simulink model "Pokus07_Display"  (Simulink 8.1)
settings: Solver=ode45  StartTime=0.0  StopTime=10.0  RelTol=1e-3
undefined symbols (not defined in the file): A, ARROW_DOWN, ARROW_LEFT, ARROW_RIGHT, ARROW_UP, ASTERISK, B, BACKSLASH, C, COLON, COMMA, CROSS, CURSOR, D, DOT, ending_column_index, ending_row_index, EQUAL, EXCLAMATION_MARK, F, framebuffer, G, GREATER_THAN, H, HEIGHT, hot, I, J, K, L, LEFT_PARENTHESES, LESS_THAN, M, MINUS, N, O, P, PERCENT, PLUS, POS_X, POS_Y, Q, QUESTION_MARK, QUOTE, R, RECTANGLE, RIGHT_PARENTHESES, S, SEMICOLON, SHARP, SLASH, SPACE, starting_column_index, starting_row_index, T, U, UNDERSCORE, V, W, WIDTH ... (+6)
libraries: dspmtrx3 x197, Common_Library x69, commutil2 x53, simulink_extras x1, dspsnks4 x1
(part 3 of 6)

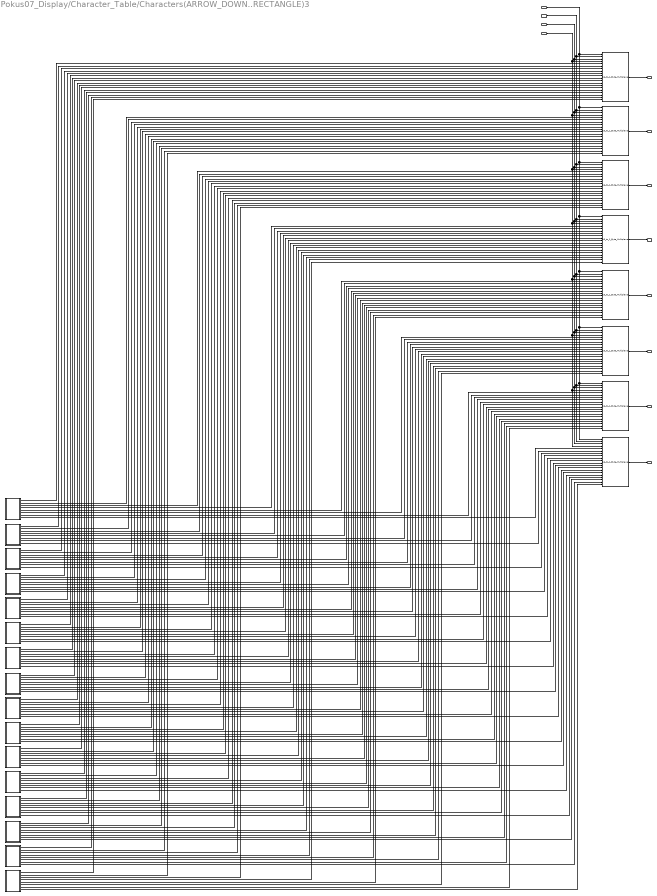
== system Pokus07_Display/Character_Table/Characters(ARROW_DOWN..RECTANGLE)3 ==
  Address_3_In(1b) : Inport
  Address_2_In(1b) : Inport  Port=2
  Address_1_In(1b) : Inport  Port=3
  Address_0_In(1b) : Inport  Port=4
  16_to_1_Byte_Multiplexer{,1..7} (8 alike) : Common_Library/Multiplexers/16_to_1_Byte_Multiplexer
  Char_ARROW_DOWN : Subsystem
  Char_ARROW_LEFT : Subsystem
  Char_ARROW_RIGHT : Subsystem
  Char_COMMA : Subsystem
  Char_CURSOR : Subsystem
  Char_DOT : Subsystem
  Char_EXCLAMATION_MARK : Subsystem
  Char_LEFT_PARENTHESES : Subsystem
  Char_PERCENT : Subsystem
  Char_QUESTION_MARK : Subsystem
  Char_QUOTE : Subsystem
  Char_RECTANGLE : Subsystem
  Char_RIGHT_PARENTHESES : Subsystem
  Char_SHARP : Subsystem
  Char_SPACE : Subsystem
  Char_UNDERSCORE : Subsystem
  Column_1(1B) : Outport
  Column_2(1B) : Outport  Port=2
  Column_3(1B) : Outport  Port=3
  Column_4(1B) : Outport  Port=4
  Column_5(1B) : Outport  Port=5
  Column_6(1B) : Outport  Port=6
  Column_7(1B) : Outport  Port=7
  Column_8(1B) : Outport  Port=8
  wires:
  Char_RECTANGLE/1(Column_1(1B)) -> 16_to_1_Byte_Multiplexer/5
  Char_CURSOR/1(Column_1(1B)) -> 16_to_1_Byte_Multiplexer/6
  Char_SPACE/1(Column_1(1B)) -> 16_to_1_Byte_Multiplexer/7
  Char_RIGHT_PARENTHESES/1(Column_1(1B)) -> 16_to_1_Byte_Multiplexer/8
  Char_LEFT_PARENTHESES/1(Column_1(1B)) -> 16_to_1_Byte_Multiplexer/9
  Char_PERCENT/1(Column_1(1B)) -> 16_to_1_Byte_Multiplexer/10
  Char_SHARP/1(Column_1(1B)) -> 16_to_1_Byte_Multiplexer/11
  Char_QUOTE/1(Column_1(1B)) -> 16_to_1_Byte_Multiplexer/12
  Char_EXCLAMATION_MARK/1(Column_1(1B)) -> 16_to_1_Byte_Multiplexer/13
  Char_QUESTION_MARK/1(Column_1(1B)) -> 16_to_1_Byte_Multiplexer/14
  Char_COMMA/1(Column_1(1B)) -> 16_to_1_Byte_Multiplexer/15
  Char_DOT/1(Column_1(1B)) -> 16_to_1_Byte_Multiplexer/16
  Char_UNDERSCORE/1(Column_1(1B)) -> 16_to_1_Byte_Multiplexer/17
  Char_ARROW_RIGHT/1(Column_1(1B)) -> 16_to_1_Byte_Multiplexer/18
  Char_ARROW_LEFT/1(Column_1(1B)) -> 16_to_1_Byte_Multiplexer/19
  Char_ARROW_DOWN/1(Column_1(1B)) -> 16_to_1_Byte_Multiplexer/20
  Char_RECTANGLE/2(Column_2(1B)) -> 16_to_1_Byte_Multiplexer1/5
  Char_ARROW_DOWN/2(Column_2(1B)) -> 16_to_1_Byte_Multiplexer1/20
  Char_ARROW_LEFT/2(Column_2(1B)) -> 16_to_1_Byte_Multiplexer1/19
  Char_ARROW_RIGHT/2(Column_2(1B)) -> 16_to_1_Byte_Multiplexer1/18
  Char_UNDERSCORE/2(Column_2(1B)) -> 16_to_1_Byte_Multiplexer1/17
  Char_DOT/2(Column_2(1B)) -> 16_to_1_Byte_Multiplexer1/16
  Char_COMMA/2(Column_2(1B)) -> 16_to_1_Byte_Multiplexer1/15
  Char_QUESTION_MARK/2(Column_2(1B)) -> 16_to_1_Byte_Multiplexer1/14
  Char_EXCLAMATION_MARK/2(Column_2(1B)) -> 16_to_1_Byte_Multiplexer1/13
  Char_QUOTE/2(Column_2(1B)) -> 16_to_1_Byte_Multiplexer1/12
  Char_SHARP/2(Column_2(1B)) -> 16_to_1_Byte_Multiplexer1/11
  Char_PERCENT/2(Column_2(1B)) -> 16_to_1_Byte_Multiplexer1/10
  Char_LEFT_PARENTHESES/2(Column_2(1B)) -> 16_to_1_Byte_Multiplexer1/9
  Char_RIGHT_PARENTHESES/2(Column_2(1B)) -> 16_to_1_Byte_Multiplexer1/8
  Char_SPACE/2(Column_2(1B)) -> 16_to_1_Byte_Multiplexer1/7
  Char_CURSOR/2(Column_2(1B)) -> 16_to_1_Byte_Multiplexer1/6
  Char_ARROW_DOWN/3(Column_3(1B)) -> 16_to_1_Byte_Multiplexer2/20
  Char_ARROW_LEFT/3(Column_3(1B)) -> 16_to_1_Byte_Multiplexer2/19
  Char_ARROW_RIGHT/3(Column_3(1B)) -> 16_to_1_Byte_Multiplexer2/18
  Char_UNDERSCORE/3(Column_3(1B)) -> 16_to_1_Byte_Multiplexer2/17
  Char_DOT/3(Column_3(1B)) -> 16_to_1_Byte_Multiplexer2/16
  Char_COMMA/3(Column_3(1B)) -> 16_to_1_Byte_Multiplexer2/15
  Char_QUESTION_MARK/3(Column_3(1B)) -> 16_to_1_Byte_Multiplexer2/14
  Char_EXCLAMATION_MARK/3(Column_3(1B)) -> 16_to_1_Byte_Multiplexer2/13
  Char_QUOTE/3(Column_3(1B)) -> 16_to_1_Byte_Multiplexer2/12
  Char_SHARP/3(Column_3(1B)) -> 16_to_1_Byte_Multiplexer2/11
  Char_PERCENT/3(Column_3(1B)) -> 16_to_1_Byte_Multiplexer2/10
  Char_LEFT_PARENTHESES/3(Column_3(1B)) -> 16_to_1_Byte_Multiplexer2/9
  Char_RIGHT_PARENTHESES/3(Column_3(1B)) -> 16_to_1_Byte_Multiplexer2/8
  Char_SPACE/3(Column_3(1B)) -> 16_to_1_Byte_Multiplexer2/7
  Char_CURSOR/3(Column_3(1B)) -> 16_to_1_Byte_Multiplexer2/6
  Char_RECTANGLE/3(Column_3(1B)) -> 16_to_1_Byte_Multiplexer2/5
  Char_ARROW_DOWN/4(Column_4(1B)) -> 16_to_1_Byte_Multiplexer3/20
  Char_ARROW_LEFT/4(Column_4(1B)) -> 16_to_1_Byte_Multiplexer3/19
  Char_ARROW_RIGHT/4(Column_4(1B)) -> 16_to_1_Byte_Multiplexer3/18
  Char_UNDERSCORE/4(Column_4(1B)) -> 16_to_1_Byte_Multiplexer3/17
  Char_DOT/4(Column_4(1B)) -> 16_to_1_Byte_Multiplexer3/16
  Char_COMMA/4(Column_4(1B)) -> 16_to_1_Byte_Multiplexer3/15
  Char_QUESTION_MARK/4(Column_4(1B)) -> 16_to_1_Byte_Multiplexer3/14
  Char_EXCLAMATION_MARK/4(Column_4(1B)) -> 16_to_1_Byte_Multiplexer3/13
  Char_QUOTE/4(Column_4(1B)) -> 16_to_1_Byte_Multiplexer3/12
  Char_SHARP/4(Column_4(1B)) -> 16_to_1_Byte_Multiplexer3/11
  Char_PERCENT/4(Column_4(1B)) -> 16_to_1_Byte_Multiplexer3/10
  Char_LEFT_PARENTHESES/4(Column_4(1B)) -> 16_to_1_Byte_Multiplexer3/9
  Char_RIGHT_PARENTHESES/4(Column_4(1B)) -> 16_to_1_Byte_Multiplexer3/8
  Char_SPACE/4(Column_4(1B)) -> 16_to_1_Byte_Multiplexer3/7
  Char_CURSOR/4(Column_4(1B)) -> 16_to_1_Byte_Multiplexer3/6
  Char_RECTANGLE/4(Column_4(1B)) -> 16_to_1_Byte_Multiplexer3/5
  Char_ARROW_DOWN/5(Column_5(1B)) -> 16_to_1_Byte_Multiplexer4/20
  Char_ARROW_LEFT/5(Column_5(1B)) -> 16_to_1_Byte_Multiplexer4/19
  Char_ARROW_RIGHT/5(Column_5(1B)) -> 16_to_1_Byte_Multiplexer4/18
  Char_UNDERSCORE/5(Column_5(1B)) -> 16_to_1_Byte_Multiplexer4/17
  Char_DOT/5(Column_5(1B)) -> 16_to_1_Byte_Multiplexer4/16
  Char_COMMA/5(Column_5(1B)) -> 16_to_1_Byte_Multiplexer4/15
  Char_EXCLAMATION_MARK/5(Column_5(1B)) -> 16_to_1_Byte_Multiplexer4/13
  Char_QUESTION_MARK/5(Column_5(1B)) -> 16_to_1_Byte_Multiplexer4/14
  Char_QUOTE/5(Column_5(1B)) -> 16_to_1_Byte_Multiplexer4/12
  Char_SHARP/5(Column_5(1B)) -> 16_to_1_Byte_Multiplexer4/11
  Char_PERCENT/5(Column_5(1B)) -> 16_to_1_Byte_Multiplexer4/10
  Char_LEFT_PARENTHESES/5(Column_5(1B)) -> 16_to_1_Byte_Multiplexer4/9
  Char_RIGHT_PARENTHESES/5(Column_5(1B)) -> 16_to_1_Byte_Multiplexer4/8
  Char_SPACE/5(Column_5(1B)) -> 16_to_1_Byte_Multiplexer4/7
  Char_CURSOR/5(Column_5(1B)) -> 16_to_1_Byte_Multiplexer4/6
  Char_RECTANGLE/5(Column_5(1B)) -> 16_to_1_Byte_Multiplexer4/5
  Char_ARROW_DOWN/6(Column_6(1B)) -> 16_to_1_Byte_Multiplexer5/20
  Char_ARROW_LEFT/6(Column_6(1B)) -> 16_to_1_Byte_Multiplexer5/19
  Char_ARROW_RIGHT/6(Column_6(1B)) -> 16_to_1_Byte_Multiplexer5/18
  Char_UNDERSCORE/6(Column_6(1B)) -> 16_to_1_Byte_Multiplexer5/17
  Char_DOT/6(Column_6(1B)) -> 16_to_1_Byte_Multiplexer5/16
  Char_COMMA/6(Column_6(1B)) -> 16_to_1_Byte_Multiplexer5/15
  Char_QUESTION_MARK/6(Column_6(1B)) -> 16_to_1_Byte_Multiplexer5/14
  Char_EXCLAMATION_MARK/6(Column_6(1B)) -> 16_to_1_Byte_Multiplexer5/13
  Char_QUOTE/6(Column_6(1B)) -> 16_to_1_Byte_Multiplexer5/12
  Char_SHARP/6(Column_6(1B)) -> 16_to_1_Byte_Multiplexer5/11
  Char_PERCENT/6(Column_6(1B)) -> 16_to_1_Byte_Multiplexer5/10
  Char_LEFT_PARENTHESES/6(Column_6(1B)) -> 16_to_1_Byte_Multiplexer5/9
  Char_RIGHT_PARENTHESES/7(Column_7(1B)) -> 16_to_1_Byte_Multiplexer6/8
  Char_RIGHT_PARENTHESES/6(Column_6(1B)) -> 16_to_1_Byte_Multiplexer5/8
  Char_SPACE/6(Column_6(1B)) -> 16_to_1_Byte_Multiplexer5/7
  Char_CURSOR/6(Column_6(1B)) -> 16_to_1_Byte_Multiplexer5/6
  Char_RECTANGLE/6(Column_6(1B)) -> 16_to_1_Byte_Multiplexer5/5
  Char_ARROW_DOWN/7(Column_7(1B)) -> 16_to_1_Byte_Multiplexer6/20
  Char_ARROW_LEFT/7(Column_7(1B)) -> 16_to_1_Byte_Multiplexer6/19
  Char_ARROW_RIGHT/7(Column_7(1B)) -> 16_to_1_Byte_Multiplexer6/18
  Char_UNDERSCORE/7(Column_7(1B)) -> 16_to_1_Byte_Multiplexer6/17
  Char_DOT/7(Column_7(1B)) -> 16_to_1_Byte_Multiplexer6/16
  Char_COMMA/7(Column_7(1B)) -> 16_to_1_Byte_Multiplexer6/15
  Char_QUESTION_MARK/7(Column_7(1B)) -> 16_to_1_Byte_Multiplexer6/14
  Char_EXCLAMATION_MARK/7(Column_7(1B)) -> 16_to_1_Byte_Multiplexer6/13
  Char_QUOTE/7(Column_7(1B)) -> 16_to_1_Byte_Multiplexer6/12
  Char_SHARP/7(Column_7(1B)) -> 16_to_1_Byte_Multiplexer6/11
  Char_PERCENT/7(Column_7(1B)) -> 16_to_1_Byte_Multiplexer6/10
  Char_LEFT_PARENTHESES/7(Column_7(1B)) -> 16_to_1_Byte_Multiplexer6/9
  Char_SPACE/7(Column_7(1B)) -> 16_to_1_Byte_Multiplexer6/7
  Char_CURSOR/7(Column_7(1B)) -> 16_to_1_Byte_Multiplexer6/6
  Char_RECTANGLE/7(Column_7(1B)) -> 16_to_1_Byte_Multiplexer6/5
  Char_ARROW_DOWN/8(Column_8(1B)) -> 16_to_1_Byte_Multiplexer7/20
  Char_ARROW_LEFT/8(Column_8(1B)) -> 16_to_1_Byte_Multiplexer7/19
  Char_ARROW_RIGHT/8(Column_8(1B)) -> 16_to_1_Byte_Multiplexer7/18
  Char_UNDERSCORE/8(Column_8(1B)) -> 16_to_1_Byte_Multiplexer7/17
  Char_DOT/8(Column_8(1B)) -> 16_to_1_Byte_Multiplexer7/16
  Char_COMMA/8(Column_8(1B)) -> 16_to_1_Byte_Multiplexer7/15
  Char_QUESTION_MARK/8(Column_8(1B)) -> 16_to_1_Byte_Multiplexer7/14
  Char_EXCLAMATION_MARK/8(Column_8(1B)) -> 16_to_1_Byte_Multiplexer7/13
  Char_QUOTE/8(Column_8(1B)) -> 16_to_1_Byte_Multiplexer7/12
  Char_SHARP/8(Column_8(1B)) -> 16_to_1_Byte_Multiplexer7/11
  Char_PERCENT/8(Column_8(1B)) -> 16_to_1_Byte_Multiplexer7/10
  Char_LEFT_PARENTHESES/8(Column_8(1B)) -> 16_to_1_Byte_Multiplexer7/9
  Char_RIGHT_PARENTHESES/8(Column_8(1B)) -> 16_to_1_Byte_Multiplexer7/8
  Char_SPACE/8(Column_8(1B)) -> 16_to_1_Byte_Multiplexer7/7
  Char_CURSOR/8(Column_8(1B)) -> 16_to_1_Byte_Multiplexer7/6
  Char_RECTANGLE/8(Column_8(1B)) -> 16_to_1_Byte_Multiplexer7/5
  16_to_1_Byte_Multiplexer/1 -> Column_1(1B)/1
  16_to_1_Byte_Multiplexer1/1 -> Column_2(1B)/1
  16_to_1_Byte_Multiplexer2/1 -> Column_3(1B)/1
  16_to_1_Byte_Multiplexer3/1 -> Column_4(1B)/1
  16_to_1_Byte_Multiplexer4/1 -> Column_5(1B)/1
  16_to_1_Byte_Multiplexer5/1 -> Column_6(1B)/1
  16_to_1_Byte_Multiplexer6/1 -> Column_7(1B)/1
  16_to_1_Byte_Multiplexer7/1 -> Column_8(1B)/1
  Address_0_In(1b)/1 -> 16_to_1_Byte_Multiplexer/4, 16_to_1_Byte_Multiplexer1/4, 16_to_1_Byte_Multiplexer2/4, 16_to_1_Byte_Multiplexer3/4, 16_to_1_Byte_Multiplexer4/4, 16_to_1_Byte_Multiplexer5/4, 16_to_1_Byte_Multiplexer6/4, 16_to_1_Byte_Multiplexer7/4
  Address_1_In(1b)/1 -> 16_to_1_Byte_Multiplexer/3, 16_to_1_Byte_Multiplexer1/3, 16_to_1_Byte_Multiplexer2/3, 16_to_1_Byte_Multiplexer3/3, 16_to_1_Byte_Multiplexer4/3, 16_to_1_Byte_Multiplexer5/3, 16_to_1_Byte_Multiplexer6/3, 16_to_1_Byte_Multiplexer7/3
  Address_2_In(1b)/1 -> 16_to_1_Byte_Multiplexer/2, 16_to_1_Byte_Multiplexer1/2, 16_to_1_Byte_Multiplexer2/2, 16_to_1_Byte_Multiplexer3/2, 16_to_1_Byte_Multiplexer4/2, 16_to_1_Byte_Multiplexer5/2, 16_to_1_Byte_Multiplexer6/2, 16_to_1_Byte_Multiplexer7/2
  Address_3_In(1b)/1 -> 16_to_1_Byte_Multiplexer/1, 16_to_1_Byte_Multiplexer1/1, 16_to_1_Byte_Multiplexer2/1, 16_to_1_Byte_Multiplexer3/1, 16_to_1_Byte_Multiplexer4/1, 16_to_1_Byte_Multiplexer5/1, 16_to_1_Byte_Multiplexer6/1, 16_to_1_Byte_Multiplexer7/1

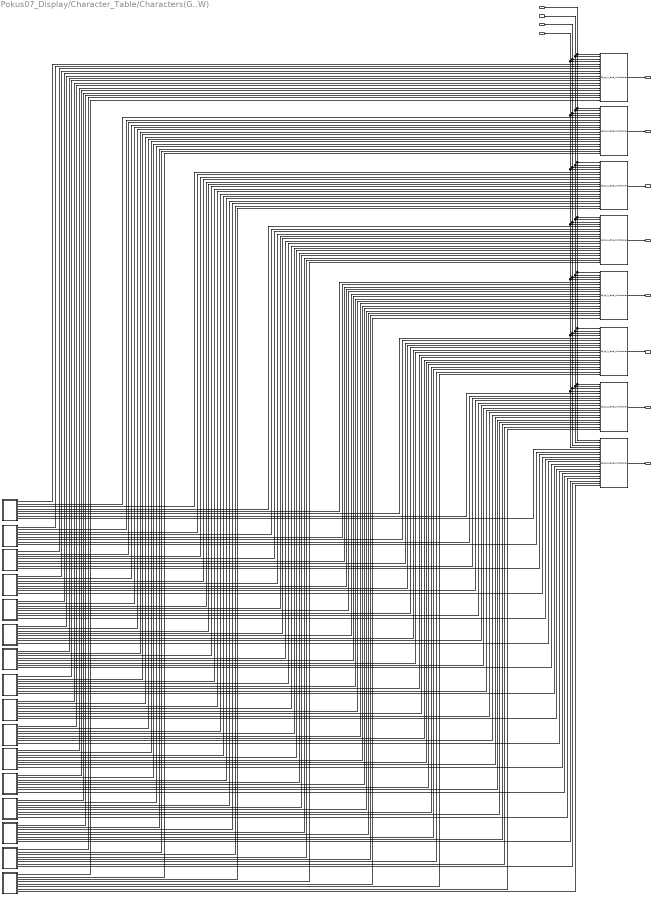
== system Pokus07_Display/Character_Table/Characters(G..W) ==
  Address_3_In(1b) : Inport
  Address_2_In(1b) : Inport  Port=2
  Address_1_In(1b) : Inport  Port=3
  Address_0_In(1b) : Inport  Port=4
  16_to_1_Byte_Multiplexer{,1..7} (8 alike) : Common_Library/Multiplexers/16_to_1_Byte_Multiplexer
  Char_G : Subsystem
  Char_H : Subsystem
  Char_I : Subsystem
  Char_J : Subsystem
  Char_K : Subsystem
  Char_L : Subsystem
  Char_M : Subsystem
  Char_N : Subsystem
  Char_O : Subsystem
  Char_P : Subsystem
  Char_R : Subsystem
  Char_S : Subsystem
  Char_T : Subsystem
  Char_U : Subsystem
  Char_V : Subsystem
  Char_W : Subsystem
  Column_1(1B) : Outport
  Column_2(1B) : Outport  Port=2
  Column_3(1B) : Outport  Port=3
  Column_4(1B) : Outport  Port=4
  Column_5(1B) : Outport  Port=5
  Column_6(1B) : Outport  Port=6
  Column_7(1B) : Outport  Port=7
  Column_8(1B) : Outport  Port=8
  wires:
  Char_W/1(Column_1(1B)) -> 16_to_1_Byte_Multiplexer/5
  Char_V/1(Column_1(1B)) -> 16_to_1_Byte_Multiplexer/6
  Char_U/1(Column_1(1B)) -> 16_to_1_Byte_Multiplexer/7
  Char_T/1(Column_1(1B)) -> 16_to_1_Byte_Multiplexer/8
  Char_S/1(Column_1(1B)) -> 16_to_1_Byte_Multiplexer/9
  Char_R/1(Column_1(1B)) -> 16_to_1_Byte_Multiplexer/10
  Char_P/1(Column_1(1B)) -> 16_to_1_Byte_Multiplexer/11
  Char_O/1(Column_1(1B)) -> 16_to_1_Byte_Multiplexer/12
  Char_N/1(Column_1(1B)) -> 16_to_1_Byte_Multiplexer/13
  Char_M/1(Column_1(1B)) -> 16_to_1_Byte_Multiplexer/14
  Char_L/1(Column_1(1B)) -> 16_to_1_Byte_Multiplexer/15
  Char_K/1(Column_1(1B)) -> 16_to_1_Byte_Multiplexer/16
  Char_J/1(Column_1(1B)) -> 16_to_1_Byte_Multiplexer/17
  Char_I/1(Column_1(1B)) -> 16_to_1_Byte_Multiplexer/18
  Char_H/1(Column_1(1B)) -> 16_to_1_Byte_Multiplexer/19
  Char_G/1(Column_1(1B)) -> 16_to_1_Byte_Multiplexer/20
  Char_W/2(Column_2(1B)) -> 16_to_1_Byte_Multiplexer1/5
  Char_G/2(Column_2(1B)) -> 16_to_1_Byte_Multiplexer1/20
  Char_H/2(Column_2(1B)) -> 16_to_1_Byte_Multiplexer1/19
  Char_I/2(Column_2(1B)) -> 16_to_1_Byte_Multiplexer1/18
  Char_J/2(Column_2(1B)) -> 16_to_1_Byte_Multiplexer1/17
  Char_K/2(Column_2(1B)) -> 16_to_1_Byte_Multiplexer1/16
  Char_L/2(Column_2(1B)) -> 16_to_1_Byte_Multiplexer1/15
  Char_M/2(Column_2(1B)) -> 16_to_1_Byte_Multiplexer1/14
  Char_N/2(Column_2(1B)) -> 16_to_1_Byte_Multiplexer1/13
  Char_O/2(Column_2(1B)) -> 16_to_1_Byte_Multiplexer1/12
  Char_P/2(Column_2(1B)) -> 16_to_1_Byte_Multiplexer1/11
  Char_R/2(Column_2(1B)) -> 16_to_1_Byte_Multiplexer1/10
  Char_S/2(Column_2(1B)) -> 16_to_1_Byte_Multiplexer1/9
  Char_T/2(Column_2(1B)) -> 16_to_1_Byte_Multiplexer1/8
  Char_U/2(Column_2(1B)) -> 16_to_1_Byte_Multiplexer1/7
  Char_V/2(Column_2(1B)) -> 16_to_1_Byte_Multiplexer1/6
  Char_G/3(Column_3(1B)) -> 16_to_1_Byte_Multiplexer2/20
  Char_H/3(Column_3(1B)) -> 16_to_1_Byte_Multiplexer2/19
  Char_I/3(Column_3(1B)) -> 16_to_1_Byte_Multiplexer2/18
  Char_J/3(Column_3(1B)) -> 16_to_1_Byte_Multiplexer2/17
  Char_K/3(Column_3(1B)) -> 16_to_1_Byte_Multiplexer2/16
  Char_L/3(Column_3(1B)) -> 16_to_1_Byte_Multiplexer2/15
  Char_M/3(Column_3(1B)) -> 16_to_1_Byte_Multiplexer2/14
  Char_N/3(Column_3(1B)) -> 16_to_1_Byte_Multiplexer2/13
  Char_O/3(Column_3(1B)) -> 16_to_1_Byte_Multiplexer2/12
  Char_P/3(Column_3(1B)) -> 16_to_1_Byte_Multiplexer2/11
  Char_R/3(Column_3(1B)) -> 16_to_1_Byte_Multiplexer2/10
  Char_S/3(Column_3(1B)) -> 16_to_1_Byte_Multiplexer2/9
  Char_T/3(Column_3(1B)) -> 16_to_1_Byte_Multiplexer2/8
  Char_U/3(Column_3(1B)) -> 16_to_1_Byte_Multiplexer2/7
  Char_V/3(Column_3(1B)) -> 16_to_1_Byte_Multiplexer2/6
  Char_W/3(Column_3(1B)) -> 16_to_1_Byte_Multiplexer2/5
  Char_G/4(Column_4(1B)) -> 16_to_1_Byte_Multiplexer3/20
  Char_H/4(Column_4(1B)) -> 16_to_1_Byte_Multiplexer3/19
  Char_I/4(Column_4(1B)) -> 16_to_1_Byte_Multiplexer3/18
  Char_J/4(Column_4(1B)) -> 16_to_1_Byte_Multiplexer3/17
  Char_K/4(Column_4(1B)) -> 16_to_1_Byte_Multiplexer3/16
  Char_L/4(Column_4(1B)) -> 16_to_1_Byte_Multiplexer3/15
  Char_M/4(Column_4(1B)) -> 16_to_1_Byte_Multiplexer3/14
  Char_N/4(Column_4(1B)) -> 16_to_1_Byte_Multiplexer3/13
  Char_O/4(Column_4(1B)) -> 16_to_1_Byte_Multiplexer3/12
  Char_P/4(Column_4(1B)) -> 16_to_1_Byte_Multiplexer3/11
  Char_R/4(Column_4(1B)) -> 16_to_1_Byte_Multiplexer3/10
  Char_S/4(Column_4(1B)) -> 16_to_1_Byte_Multiplexer3/9
  Char_T/4(Column_4(1B)) -> 16_to_1_Byte_Multiplexer3/8
  Char_U/4(Column_4(1B)) -> 16_to_1_Byte_Multiplexer3/7
  Char_V/4(Column_4(1B)) -> 16_to_1_Byte_Multiplexer3/6
  Char_W/4(Column_4(1B)) -> 16_to_1_Byte_Multiplexer3/5
  Char_G/5(Column_5(1B)) -> 16_to_1_Byte_Multiplexer4/20
  Char_H/5(Column_5(1B)) -> 16_to_1_Byte_Multiplexer4/19
  Char_I/5(Column_5(1B)) -> 16_to_1_Byte_Multiplexer4/18
  Char_J/5(Column_5(1B)) -> 16_to_1_Byte_Multiplexer4/17
  Char_K/5(Column_5(1B)) -> 16_to_1_Byte_Multiplexer4/16
  Char_L/5(Column_5(1B)) -> 16_to_1_Byte_Multiplexer4/15
  Char_N/5(Column_5(1B)) -> 16_to_1_Byte_Multiplexer4/13
  Char_M/5(Column_5(1B)) -> 16_to_1_Byte_Multiplexer4/14
  Char_O/5(Column_5(1B)) -> 16_to_1_Byte_Multiplexer4/12
  Char_P/5(Column_5(1B)) -> 16_to_1_Byte_Multiplexer4/11
  Char_R/5(Column_5(1B)) -> 16_to_1_Byte_Multiplexer4/10
  Char_S/5(Column_5(1B)) -> 16_to_1_Byte_Multiplexer4/9
  Char_T/5(Column_5(1B)) -> 16_to_1_Byte_Multiplexer4/8
  Char_U/5(Column_5(1B)) -> 16_to_1_Byte_Multiplexer4/7
  Char_V/5(Column_5(1B)) -> 16_to_1_Byte_Multiplexer4/6
  Char_W/5(Column_5(1B)) -> 16_to_1_Byte_Multiplexer4/5
  Char_G/6(Column_6(1B)) -> 16_to_1_Byte_Multiplexer5/20
  Char_H/6(Column_6(1B)) -> 16_to_1_Byte_Multiplexer5/19
  Char_I/6(Column_6(1B)) -> 16_to_1_Byte_Multiplexer5/18
  Char_J/6(Column_6(1B)) -> 16_to_1_Byte_Multiplexer5/17
  Char_K/6(Column_6(1B)) -> 16_to_1_Byte_Multiplexer5/16
  Char_L/6(Column_6(1B)) -> 16_to_1_Byte_Multiplexer5/15
  Char_M/6(Column_6(1B)) -> 16_to_1_Byte_Multiplexer5/14
  Char_N/6(Column_6(1B)) -> 16_to_1_Byte_Multiplexer5/13
  Char_O/6(Column_6(1B)) -> 16_to_1_Byte_Multiplexer5/12
  Char_P/6(Column_6(1B)) -> 16_to_1_Byte_Multiplexer5/11
  Char_R/6(Column_6(1B)) -> 16_to_1_Byte_Multiplexer5/10
  Char_S/6(Column_6(1B)) -> 16_to_1_Byte_Multiplexer5/9
  Char_T/7(Column_7(1B)) -> 16_to_1_Byte_Multiplexer6/8
  Char_T/6(Column_6(1B)) -> 16_to_1_Byte_Multiplexer5/8
  Char_U/6(Column_6(1B)) -> 16_to_1_Byte_Multiplexer5/7
  Char_V/6(Column_6(1B)) -> 16_to_1_Byte_Multiplexer5/6
  Char_W/6(Column_6(1B)) -> 16_to_1_Byte_Multiplexer5/5
  Char_G/7(Column_7(1B)) -> 16_to_1_Byte_Multiplexer6/20
  Char_H/7(Column_7(1B)) -> 16_to_1_Byte_Multiplexer6/19
  Char_I/7(Column_7(1B)) -> 16_to_1_Byte_Multiplexer6/18
  Char_J/7(Column_7(1B)) -> 16_to_1_Byte_Multiplexer6/17
  Char_K/7(Column_7(1B)) -> 16_to_1_Byte_Multiplexer6/16
  Char_L/7(Column_7(1B)) -> 16_to_1_Byte_Multiplexer6/15
  Char_M/7(Column_7(1B)) -> 16_to_1_Byte_Multiplexer6/14
  Char_N/7(Column_7(1B)) -> 16_to_1_Byte_Multiplexer6/13
  Char_O/7(Column_7(1B)) -> 16_to_1_Byte_Multiplexer6/12
  Char_P/7(Column_7(1B)) -> 16_to_1_Byte_Multiplexer6/11
  Char_R/7(Column_7(1B)) -> 16_to_1_Byte_Multiplexer6/10
  Char_S/7(Column_7(1B)) -> 16_to_1_Byte_Multiplexer6/9
  Char_U/7(Column_7(1B)) -> 16_to_1_Byte_Multiplexer6/7
  Char_V/7(Column_7(1B)) -> 16_to_1_Byte_Multiplexer6/6
  Char_W/7(Column_7(1B)) -> 16_to_1_Byte_Multiplexer6/5
  Char_G/8(Column_8(1B)) -> 16_to_1_Byte_Multiplexer7/20
  Char_H/8(Column_8(1B)) -> 16_to_1_Byte_Multiplexer7/19
  Char_I/8(Column_8(1B)) -> 16_to_1_Byte_Multiplexer7/18
  Char_J/8(Column_8(1B)) -> 16_to_1_Byte_Multiplexer7/17
  Char_K/8(Column_8(1B)) -> 16_to_1_Byte_Multiplexer7/16
  Char_L/8(Column_8(1B)) -> 16_to_1_Byte_Multiplexer7/15
  Char_M/8(Column_8(1B)) -> 16_to_1_Byte_Multiplexer7/14
  Char_N/8(Column_8(1B)) -> 16_to_1_Byte_Multiplexer7/13
  Char_O/8(Column_8(1B)) -> 16_to_1_Byte_Multiplexer7/12
  Char_P/8(Column_8(1B)) -> 16_to_1_Byte_Multiplexer7/11
  Char_R/8(Column_8(1B)) -> 16_to_1_Byte_Multiplexer7/10
  Char_S/8(Column_8(1B)) -> 16_to_1_Byte_Multiplexer7/9
  Char_T/8(Column_8(1B)) -> 16_to_1_Byte_Multiplexer7/8
  Char_U/8(Column_8(1B)) -> 16_to_1_Byte_Multiplexer7/7
  Char_V/8(Column_8(1B)) -> 16_to_1_Byte_Multiplexer7/6
  Char_W/8(Column_8(1B)) -> 16_to_1_Byte_Multiplexer7/5
  16_to_1_Byte_Multiplexer/1 -> Column_1(1B)/1
  16_to_1_Byte_Multiplexer1/1 -> Column_2(1B)/1
  16_to_1_Byte_Multiplexer2/1 -> Column_3(1B)/1
  16_to_1_Byte_Multiplexer3/1 -> Column_4(1B)/1
  16_to_1_Byte_Multiplexer4/1 -> Column_5(1B)/1
  16_to_1_Byte_Multiplexer5/1 -> Column_6(1B)/1
  16_to_1_Byte_Multiplexer6/1 -> Column_7(1B)/1
  16_to_1_Byte_Multiplexer7/1 -> Column_8(1B)/1
  Address_0_In(1b)/1 -> 16_to_1_Byte_Multiplexer/4, 16_to_1_Byte_Multiplexer1/4, 16_to_1_Byte_Multiplexer2/4, 16_to_1_Byte_Multiplexer3/4, 16_to_1_Byte_Multiplexer4/4, 16_to_1_Byte_Multiplexer5/4, 16_to_1_Byte_Multiplexer6/4, 16_to_1_Byte_Multiplexer7/4
  Address_1_In(1b)/1 -> 16_to_1_Byte_Multiplexer/3, 16_to_1_Byte_Multiplexer1/3, 16_to_1_Byte_Multiplexer2/3, 16_to_1_Byte_Multiplexer3/3, 16_to_1_Byte_Multiplexer4/3, 16_to_1_Byte_Multiplexer5/3, 16_to_1_Byte_Multiplexer6/3, 16_to_1_Byte_Multiplexer7/3
  Address_2_In(1b)/1 -> 16_to_1_Byte_Multiplexer/2, 16_to_1_Byte_Multiplexer1/2, 16_to_1_Byte_Multiplexer2/2, 16_to_1_Byte_Multiplexer3/2, 16_to_1_Byte_Multiplexer4/2, 16_to_1_Byte_Multiplexer5/2, 16_to_1_Byte_Multiplexer6/2, 16_to_1_Byte_Multiplexer7/2
  Address_3_In(1b)/1 -> 16_to_1_Byte_Multiplexer/1, 16_to_1_Byte_Multiplexer1/1, 16_to_1_Byte_Multiplexer2/1, 16_to_1_Byte_Multiplexer3/1, 16_to_1_Byte_Multiplexer4/1, 16_to_1_Byte_Multiplexer5/1, 16_to_1_Byte_Multiplexer6/1, 16_to_1_Byte_Multiplexer7/1

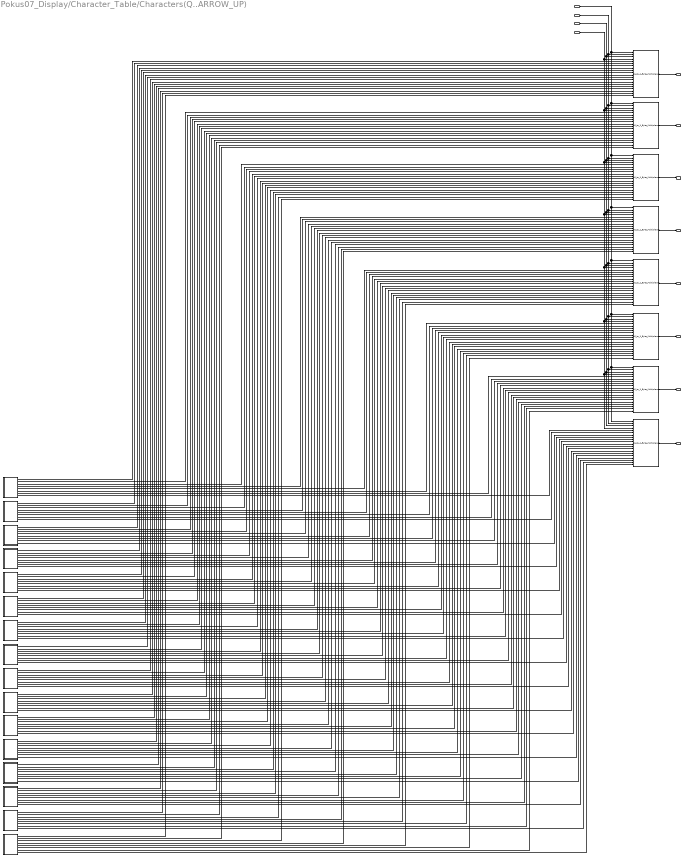
== system Pokus07_Display/Character_Table/Characters(Q..ARROW_UP) ==
  Address_3_In(1b) : Inport
  Address_2_In(1b) : Inport  Port=2
  Address_1_In(1b) : Inport  Port=3
  Address_0_In(1b) : Inport  Port=4
  16_to_1_Byte_Multiplexer{,1..7} (8 alike) : Common_Library/Multiplexers/16_to_1_Byte_Multiplexer
  Char_ARROW_UP : Subsystem
  Char_ASTERISK : Subsystem
  Char_BACKSLASH : Subsystem
  Char_COLON : Subsystem
  Char_CROSS : Subsystem
  Char_EQUAL : Subsystem
  Char_GREATER_THAN : Subsystem
  Char_LESS_THAN : Subsystem
  Char_MINUS : Subsystem
  Char_PLUS : Subsystem
  Char_Q : Subsystem
  Char_SEMICOLON : Subsystem
  Char_SLASH : Subsystem
  Char_X : Subsystem
  Char_Y : Subsystem
  Char_Z : Subsystem
  Column_1(1B) : Outport
  Column_2(1B) : Outport  Port=2
  Column_3(1B) : Outport  Port=3
  Column_4(1B) : Outport  Port=4
  Column_5(1B) : Outport  Port=5
  Column_6(1B) : Outport  Port=6
  Column_7(1B) : Outport  Port=7
  Column_8(1B) : Outport  Port=8
  wires:
  Char_ARROW_UP/1(Column_1(1B)) -> 16_to_1_Byte_Multiplexer/5
  Char_GREATER_THAN/1(Column_1(1B)) -> 16_to_1_Byte_Multiplexer/6
  Char_LESS_THAN/1(Column_1(1B)) -> 16_to_1_Byte_Multiplexer/7
  Char_EQUAL/1(Column_1(1B)) -> 16_to_1_Byte_Multiplexer/8
  Char_BACKSLASH/1(Column_1(1B)) -> 16_to_1_Byte_Multiplexer/9
  Char_SLASH/1(Column_1(1B)) -> 16_to_1_Byte_Multiplexer/10
  Char_SEMICOLON/1(Column_1(1B)) -> 16_to_1_Byte_Multiplexer/11
  Char_COLON/1(Column_1(1B)) -> 16_to_1_Byte_Multiplexer/12
  Char_ASTERISK/1(Column_1(1B)) -> 16_to_1_Byte_Multiplexer/13
  Char_CROSS/1(Column_1(1B)) -> 16_to_1_Byte_Multiplexer/14
  Char_MINUS/1(Column_1(1B)) -> 16_to_1_Byte_Multiplexer/15
  Char_PLUS/1(Column_1(1B)) -> 16_to_1_Byte_Multiplexer/16
  Char_Z/1(Column_1(1B)) -> 16_to_1_Byte_Multiplexer/17
  Char_Y/1(Column_1(1B)) -> 16_to_1_Byte_Multiplexer/18
  Char_X/1(Column_1(1B)) -> 16_to_1_Byte_Multiplexer/19
  Char_Q/1(Column_1(1B)) -> 16_to_1_Byte_Multiplexer/20
  Char_ARROW_UP/2(Column_2(1B)) -> 16_to_1_Byte_Multiplexer1/5
  Char_Q/2(Column_2(1B)) -> 16_to_1_Byte_Multiplexer1/20
  Char_X/2(Column_2(1B)) -> 16_to_1_Byte_Multiplexer1/19
  Char_Y/2(Column_2(1B)) -> 16_to_1_Byte_Multiplexer1/18
  Char_Z/2(Column_2(1B)) -> 16_to_1_Byte_Multiplexer1/17
  Char_PLUS/2(Column_2(1B)) -> 16_to_1_Byte_Multiplexer1/16
  Char_MINUS/2(Column_2(1B)) -> 16_to_1_Byte_Multiplexer1/15
  Char_CROSS/2(Column_2(1B)) -> 16_to_1_Byte_Multiplexer1/14
  Char_ASTERISK/2(Column_2(1B)) -> 16_to_1_Byte_Multiplexer1/13
  Char_COLON/2(Column_2(1B)) -> 16_to_1_Byte_Multiplexer1/12
  Char_SEMICOLON/2(Column_2(1B)) -> 16_to_1_Byte_Multiplexer1/11
  Char_SLASH/2(Column_2(1B)) -> 16_to_1_Byte_Multiplexer1/10
  Char_BACKSLASH/2(Column_2(1B)) -> 16_to_1_Byte_Multiplexer1/9
  Char_EQUAL/2(Column_2(1B)) -> 16_to_1_Byte_Multiplexer1/8
  Char_LESS_THAN/2(Column_2(1B)) -> 16_to_1_Byte_Multiplexer1/7
  Char_GREATER_THAN/2(Column_2(1B)) -> 16_to_1_Byte_Multiplexer1/6
  Char_Q/3(Column_3(1B)) -> 16_to_1_Byte_Multiplexer2/20
  Char_X/3(Column_3(1B)) -> 16_to_1_Byte_Multiplexer2/19
  Char_Y/3(Column_3(1B)) -> 16_to_1_Byte_Multiplexer2/18
  Char_Z/3(Column_3(1B)) -> 16_to_1_Byte_Multiplexer2/17
  Char_PLUS/3(Column_3(1B)) -> 16_to_1_Byte_Multiplexer2/16
  Char_MINUS/3(Column_3(1B)) -> 16_to_1_Byte_Multiplexer2/15
  Char_CROSS/3(Column_3(1B)) -> 16_to_1_Byte_Multiplexer2/14
  Char_ASTERISK/3(Column_3(1B)) -> 16_to_1_Byte_Multiplexer2/13
  Char_COLON/3(Column_3(1B)) -> 16_to_1_Byte_Multiplexer2/12
  Char_SEMICOLON/3(Column_3(1B)) -> 16_to_1_Byte_Multiplexer2/11
  Char_SLASH/3(Column_3(1B)) -> 16_to_1_Byte_Multiplexer2/10
  Char_BACKSLASH/3(Column_3(1B)) -> 16_to_1_Byte_Multiplexer2/9
  Char_EQUAL/3(Column_3(1B)) -> 16_to_1_Byte_Multiplexer2/8
  Char_LESS_THAN/3(Column_3(1B)) -> 16_to_1_Byte_Multiplexer2/7
  Char_GREATER_THAN/3(Column_3(1B)) -> 16_to_1_Byte_Multiplexer2/6
  Char_ARROW_UP/3(Column_3(1B)) -> 16_to_1_Byte_Multiplexer2/5
  Char_Q/4(Column_4(1B)) -> 16_to_1_Byte_Multiplexer3/20
  Char_X/4(Column_4(1B)) -> 16_to_1_Byte_Multiplexer3/19
  Char_Y/4(Column_4(1B)) -> 16_to_1_Byte_Multiplexer3/18
  Char_Z/4(Column_4(1B)) -> 16_to_1_Byte_Multiplexer3/17
  Char_PLUS/4(Column_4(1B)) -> 16_to_1_Byte_Multiplexer3/16
  Char_MINUS/4(Column_4(1B)) -> 16_to_1_Byte_Multiplexer3/15
  Char_CROSS/4(Column_4(1B)) -> 16_to_1_Byte_Multiplexer3/14
  Char_ASTERISK/4(Column_4(1B)) -> 16_to_1_Byte_Multiplexer3/13
  Char_COLON/4(Column_4(1B)) -> 16_to_1_Byte_Multiplexer3/12
  Char_SEMICOLON/4(Column_4(1B)) -> 16_to_1_Byte_Multiplexer3/11
  Char_SLASH/4(Column_4(1B)) -> 16_to_1_Byte_Multiplexer3/10
  Char_BACKSLASH/4(Column_4(1B)) -> 16_to_1_Byte_Multiplexer3/9
  Char_EQUAL/4(Column_4(1B)) -> 16_to_1_Byte_Multiplexer3/8
  Char_LESS_THAN/4(Column_4(1B)) -> 16_to_1_Byte_Multiplexer3/7
  Char_GREATER_THAN/4(Column_4(1B)) -> 16_to_1_Byte_Multiplexer3/6
  Char_ARROW_UP/4(Column_4(1B)) -> 16_to_1_Byte_Multiplexer3/5
  Char_Q/5(Column_5(1B)) -> 16_to_1_Byte_Multiplexer4/20
  Char_X/5(Column_5(1B)) -> 16_to_1_Byte_Multiplexer4/19
  Char_Y/5(Column_5(1B)) -> 16_to_1_Byte_Multiplexer4/18
  Char_Z/5(Column_5(1B)) -> 16_to_1_Byte_Multiplexer4/17
  Char_PLUS/5(Column_5(1B)) -> 16_to_1_Byte_Multiplexer4/16
  Char_MINUS/5(Column_5(1B)) -> 16_to_1_Byte_Multiplexer4/15
  Char_ASTERISK/5(Column_5(1B)) -> 16_to_1_Byte_Multiplexer4/13
  Char_CROSS/5(Column_5(1B)) -> 16_to_1_Byte_Multiplexer4/14
  Char_COLON/5(Column_5(1B)) -> 16_to_1_Byte_Multiplexer4/12
  Char_SEMICOLON/5(Column_5(1B)) -> 16_to_1_Byte_Multiplexer4/11
  Char_SLASH/5(Column_5(1B)) -> 16_to_1_Byte_Multiplexer4/10
  Char_BACKSLASH/5(Column_5(1B)) -> 16_to_1_Byte_Multiplexer4/9
  Char_EQUAL/5(Column_5(1B)) -> 16_to_1_Byte_Multiplexer4/8
  Char_LESS_THAN/5(Column_5(1B)) -> 16_to_1_Byte_Multiplexer4/7
  Char_GREATER_THAN/5(Column_5(1B)) -> 16_to_1_Byte_Multiplexer4/6
  Char_ARROW_UP/5(Column_5(1B)) -> 16_to_1_Byte_Multiplexer4/5
  Char_Q/6(Column_6(1B)) -> 16_to_1_Byte_Multiplexer5/20
  Char_X/6(Column_6(1B)) -> 16_to_1_Byte_Multiplexer5/19
  Char_Y/6(Column_6(1B)) -> 16_to_1_Byte_Multiplexer5/18
  Char_Z/6(Column_6(1B)) -> 16_to_1_Byte_Multiplexer5/17
  Char_PLUS/6(Column_6(1B)) -> 16_to_1_Byte_Multiplexer5/16
  Char_MINUS/6(Column_6(1B)) -> 16_to_1_Byte_Multiplexer5/15
  Char_CROSS/6(Column_6(1B)) -> 16_to_1_Byte_Multiplexer5/14
  Char_ASTERISK/6(Column_6(1B)) -> 16_to_1_Byte_Multiplexer5/13
  Char_COLON/6(Column_6(1B)) -> 16_to_1_Byte_Multiplexer5/12
  Char_SEMICOLON/6(Column_6(1B)) -> 16_to_1_Byte_Multiplexer5/11
  Char_SLASH/6(Column_6(1B)) -> 16_to_1_Byte_Multiplexer5/10
  Char_BACKSLASH/6(Column_6(1B)) -> 16_to_1_Byte_Multiplexer5/9
  Char_EQUAL/7(Column_7(1B)) -> 16_to_1_Byte_Multiplexer6/8
  Char_EQUAL/6(Column_6(1B)) -> 16_to_1_Byte_Multiplexer5/8
  Char_LESS_THAN/6(Column_6(1B)) -> 16_to_1_Byte_Multiplexer5/7
  Char_GREATER_THAN/6(Column_6(1B)) -> 16_to_1_Byte_Multiplexer5/6
  Char_ARROW_UP/6(Column_6(1B)) -> 16_to_1_Byte_Multiplexer5/5
  Char_Q/7(Column_7(1B)) -> 16_to_1_Byte_Multiplexer6/20
  Char_X/7(Column_7(1B)) -> 16_to_1_Byte_Multiplexer6/19
  Char_Y/7(Column_7(1B)) -> 16_to_1_Byte_Multiplexer6/18
  Char_Z/7(Column_7(1B)) -> 16_to_1_Byte_Multiplexer6/17
  Char_PLUS/7(Column_7(1B)) -> 16_to_1_Byte_Multiplexer6/16
  Char_MINUS/7(Column_7(1B)) -> 16_to_1_Byte_Multiplexer6/15
  Char_CROSS/7(Column_7(1B)) -> 16_to_1_Byte_Multiplexer6/14
  Char_ASTERISK/7(Column_7(1B)) -> 16_to_1_Byte_Multiplexer6/13
  Char_COLON/7(Column_7(1B)) -> 16_to_1_Byte_Multiplexer6/12
  Char_SEMICOLON/7(Column_7(1B)) -> 16_to_1_Byte_Multiplexer6/11
  Char_SLASH/7(Column_7(1B)) -> 16_to_1_Byte_Multiplexer6/10
  Char_BACKSLASH/7(Column_7(1B)) -> 16_to_1_Byte_Multiplexer6/9
  Char_LESS_THAN/7(Column_7(1B)) -> 16_to_1_Byte_Multiplexer6/7
  Char_GREATER_THAN/7(Column_7(1B)) -> 16_to_1_Byte_Multiplexer6/6
  Char_ARROW_UP/7(Column_7(1B)) -> 16_to_1_Byte_Multiplexer6/5
  Char_Q/8(Column_8(1B)) -> 16_to_1_Byte_Multiplexer7/20
  Char_X/8(Column_8(1B)) -> 16_to_1_Byte_Multiplexer7/19
  Char_Y/8(Column_8(1B)) -> 16_to_1_Byte_Multiplexer7/18
  Char_Z/8(Column_8(1B)) -> 16_to_1_Byte_Multiplexer7/17
  Char_PLUS/8(Column_8(1B)) -> 16_to_1_Byte_Multiplexer7/16
  Char_MINUS/8(Column_8(1B)) -> 16_to_1_Byte_Multiplexer7/15
  Char_CROSS/8(Column_8(1B)) -> 16_to_1_Byte_Multiplexer7/14
  Char_ASTERISK/8(Column_8(1B)) -> 16_to_1_Byte_Multiplexer7/13
  Char_COLON/8(Column_8(1B)) -> 16_to_1_Byte_Multiplexer7/12
  Char_SEMICOLON/8(Column_8(1B)) -> 16_to_1_Byte_Multiplexer7/11
  Char_SLASH/8(Column_8(1B)) -> 16_to_1_Byte_Multiplexer7/10
  Char_BACKSLASH/8(Column_8(1B)) -> 16_to_1_Byte_Multiplexer7/9
  Char_EQUAL/8(Column_8(1B)) -> 16_to_1_Byte_Multiplexer7/8
  Char_LESS_THAN/8(Column_8(1B)) -> 16_to_1_Byte_Multiplexer7/7
  Char_GREATER_THAN/8(Column_8(1B)) -> 16_to_1_Byte_Multiplexer7/6
  Char_ARROW_UP/8(Column_8(1B)) -> 16_to_1_Byte_Multiplexer7/5
  16_to_1_Byte_Multiplexer/1 -> Column_1(1B)/1
  16_to_1_Byte_Multiplexer1/1 -> Column_2(1B)/1
  16_to_1_Byte_Multiplexer2/1 -> Column_3(1B)/1
  16_to_1_Byte_Multiplexer3/1 -> Column_4(1B)/1
  16_to_1_Byte_Multiplexer4/1 -> Column_5(1B)/1
  16_to_1_Byte_Multiplexer5/1 -> Column_6(1B)/1
  16_to_1_Byte_Multiplexer6/1 -> Column_7(1B)/1
  16_to_1_Byte_Multiplexer7/1 -> Column_8(1B)/1
  Address_0_In(1b)/1 -> 16_to_1_Byte_Multiplexer/4, 16_to_1_Byte_Multiplexer1/4, 16_to_1_Byte_Multiplexer2/4, 16_to_1_Byte_Multiplexer3/4, 16_to_1_Byte_Multiplexer4/4, 16_to_1_Byte_Multiplexer5/4, 16_to_1_Byte_Multiplexer6/4, 16_to_1_Byte_Multiplexer7/4
  Address_1_In(1b)/1 -> 16_to_1_Byte_Multiplexer/3, 16_to_1_Byte_Multiplexer1/3, 16_to_1_Byte_Multiplexer2/3, 16_to_1_Byte_Multiplexer3/3, 16_to_1_Byte_Multiplexer4/3, 16_to_1_Byte_Multiplexer5/3, 16_to_1_Byte_Multiplexer6/3, 16_to_1_Byte_Multiplexer7/3
  Address_2_In(1b)/1 -> 16_to_1_Byte_Multiplexer/2, 16_to_1_Byte_Multiplexer1/2, 16_to_1_Byte_Multiplexer2/2, 16_to_1_Byte_Multiplexer3/2, 16_to_1_Byte_Multiplexer4/2, 16_to_1_Byte_Multiplexer5/2, 16_to_1_Byte_Multiplexer6/2, 16_to_1_Byte_Multiplexer7/2
  Address_3_In(1b)/1 -> 16_to_1_Byte_Multiplexer/1, 16_to_1_Byte_Multiplexer1/1, 16_to_1_Byte_Multiplexer2/1, 16_to_1_Byte_Multiplexer3/1, 16_to_1_Byte_Multiplexer4/1, 16_to_1_Byte_Multiplexer5/1, 16_to_1_Byte_Multiplexer6/1, 16_to_1_Byte_Multiplexer7/1

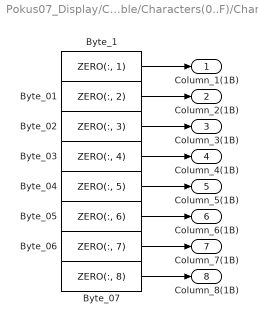
== system Pokus07_Display/Character_Table/Characters(0..F)/Char_0 ==
  Byte_01 : Constant  Value=ZERO(:, 2)  OutDataTypeStr=uint8
  Byte_02 : Constant  Value=ZERO(:, 3)  OutDataTypeStr=uint8
  Byte_03 : Constant  Value=ZERO(:, 4)  OutDataTypeStr=uint8
  Byte_04 : Constant  Value=ZERO(:, 5)  OutDataTypeStr=uint8
  Byte_05 : Constant  Value=ZERO(:, 6)  OutDataTypeStr=uint8
  Byte_06 : Constant  Value=ZERO(:, 7)  OutDataTypeStr=uint8
  Byte_07 : Constant  Value=ZERO(:, 8)  OutDataTypeStr=uint8
  Byte_1 : Constant  Value=ZERO(:, 1)  OutDataTypeStr=uint8
  Column_1(1B) : Outport
  Column_2(1B) : Outport  Port=2
  Column_3(1B) : Outport  Port=3
  Column_4(1B) : Outport  Port=4
  Column_5(1B) : Outport  Port=5
  Column_6(1B) : Outport  Port=6
  Column_7(1B) : Outport  Port=7
  Column_8(1B) : Outport  Port=8
  wires:
  Byte_05/1 -> Column_6(1B)/1
  Byte_04/1 -> Column_5(1B)/1
  Byte_01/1 -> Column_2(1B)/1
  Byte_07/1 -> Column_8(1B)/1
  Byte_03/1 -> Column_4(1B)/1
  Byte_06/1 -> Column_7(1B)/1
  Byte_1/1 -> Column_1(1B)/1
  Byte_02/1 -> Column_3(1B)/1

== system Pokus07_Display/Character_Table/Characters(0..F)/Char_1 ==
  Byte_01 : Constant  Value=char(:, 2, 1)  OutDataTypeStr=uint8
  Byte_02 : Constant  Value=char(:, 3, 1)  OutDataTypeStr=uint8
  Byte_03 : Constant  Value=char(:, 4, 1)  OutDataTypeStr=uint8
  Byte_04 : Constant  Value=char(:, 5, 1)  OutDataTypeStr=uint8
  Byte_05 : Constant  Value=char(:, 6, 1)  OutDataTypeStr=uint8
  Byte_06 : Constant  Value=char(:, 7, 1)  OutDataTypeStr=uint8
  Byte_07 : Constant  Value=char(:, 8, 1)  OutDataTypeStr=uint8
  Byte_1 : Constant  Value=char(:, 1, 1)  OutDataTypeStr=uint8
  Column_1(1B) : Outport
  Column_2(1B) : Outport  Port=2
  Column_3(1B) : Outport  Port=3
  Column_4(1B) : Outport  Port=4
  Column_5(1B) : Outport  Port=5
  Column_6(1B) : Outport  Port=6
  Column_7(1B) : Outport  Port=7
  Column_8(1B) : Outport  Port=8
  wires:
  Byte_05/1 -> Column_6(1B)/1
  Byte_04/1 -> Column_5(1B)/1
  Byte_01/1 -> Column_2(1B)/1
  Byte_07/1 -> Column_8(1B)/1
  Byte_03/1 -> Column_4(1B)/1
  Byte_06/1 -> Column_7(1B)/1
  Byte_1/1 -> Column_1(1B)/1
  Byte_02/1 -> Column_3(1B)/1

== system Pokus07_Display/Character_Table/Characters(0..F)/Char_2 ==
  Byte_01 : Constant  Value=char(:, 2, 2)  OutDataTypeStr=uint8
  Byte_02 : Constant  Value=char(:, 3, 2)  OutDataTypeStr=uint8
  Byte_03 : Constant  Value=char(:, 4, 2)  OutDataTypeStr=uint8
  Byte_04 : Constant  Value=char(:, 5, 2)  OutDataTypeStr=uint8
  Byte_05 : Constant  Value=char(:, 6, 2)  OutDataTypeStr=uint8
  Byte_06 : Constant  Value=char(:, 7, 2)  OutDataTypeStr=uint8
  Byte_07 : Constant  Value=char(:, 8, 2)  OutDataTypeStr=uint8
  Byte_1 : Constant  Value=char(:, 1, 2)  OutDataTypeStr=uint8
  Column_1(1B) : Outport
  Column_2(1B) : Outport  Port=2
  Column_3(1B) : Outport  Port=3
  Column_4(1B) : Outport  Port=4
  Column_5(1B) : Outport  Port=5
  Column_6(1B) : Outport  Port=6
  Column_7(1B) : Outport  Port=7
  Column_8(1B) : Outport  Port=8
  wires:
  Byte_05/1 -> Column_6(1B)/1
  Byte_04/1 -> Column_5(1B)/1
  Byte_01/1 -> Column_2(1B)/1
  Byte_07/1 -> Column_8(1B)/1
  Byte_03/1 -> Column_4(1B)/1
  Byte_06/1 -> Column_7(1B)/1
  Byte_1/1 -> Column_1(1B)/1
  Byte_02/1 -> Column_3(1B)/1

== system Pokus07_Display/Character_Table/Characters(0..F)/Char_3 ==
  Byte_01 : Constant  Value=char(:, 2, 3)  OutDataTypeStr=uint8
  Byte_02 : Constant  Value=char(:, 3, 3)  OutDataTypeStr=uint8
  Byte_03 : Constant  Value=char(:, 4, 3)  OutDataTypeStr=uint8
  Byte_04 : Constant  Value=char(:, 5, 3)  OutDataTypeStr=uint8
  Byte_05 : Constant  Value=char(:, 6, 3)  OutDataTypeStr=uint8
  Byte_06 : Constant  Value=char(:, 7, 3)  OutDataTypeStr=uint8
  Byte_07 : Constant  Value=char(:, 8, 3)  OutDataTypeStr=uint8
  Byte_1 : Constant  Value=char(:, 1, 3)  OutDataTypeStr=uint8
  Column_1(1B) : Outport
  Column_2(1B) : Outport  Port=2
  Column_3(1B) : Outport  Port=3
  Column_4(1B) : Outport  Port=4
  Column_5(1B) : Outport  Port=5
  Column_6(1B) : Outport  Port=6
  Column_7(1B) : Outport  Port=7
  Column_8(1B) : Outport  Port=8
  wires:
  Byte_05/1 -> Column_6(1B)/1
  Byte_04/1 -> Column_5(1B)/1
  Byte_01/1 -> Column_2(1B)/1
  Byte_07/1 -> Column_8(1B)/1
  Byte_03/1 -> Column_4(1B)/1
  Byte_06/1 -> Column_7(1B)/1
  Byte_1/1 -> Column_1(1B)/1
  Byte_02/1 -> Column_3(1B)/1

== system Pokus07_Display/Character_Table/Characters(0..F)/Char_4 ==
  Byte_01 : Constant  Value=char(:, 2, 4)  OutDataTypeStr=uint8
  Byte_02 : Constant  Value=char(:, 3, 4)  OutDataTypeStr=uint8
  Byte_03 : Constant  Value=char(:, 4, 4)  OutDataTypeStr=uint8
  Byte_04 : Constant  Value=char(:, 5, 4)  OutDataTypeStr=uint8
  Byte_05 : Constant  Value=char(:, 6, 4)  OutDataTypeStr=uint8
  Byte_06 : Constant  Value=char(:, 7, 4)  OutDataTypeStr=uint8
  Byte_07 : Constant  Value=char(:, 8, 4)  OutDataTypeStr=uint8
  Byte_1 : Constant  Value=char(:, 1, 4)  OutDataTypeStr=uint8
  Column_1(1B) : Outport
  Column_2(1B) : Outport  Port=2
  Column_3(1B) : Outport  Port=3
  Column_4(1B) : Outport  Port=4
  Column_5(1B) : Outport  Port=5
  Column_6(1B) : Outport  Port=6
  Column_7(1B) : Outport  Port=7
  Column_8(1B) : Outport  Port=8
  wires:
  Byte_05/1 -> Column_6(1B)/1
  Byte_04/1 -> Column_5(1B)/1
  Byte_01/1 -> Column_2(1B)/1
  Byte_07/1 -> Column_8(1B)/1
  Byte_03/1 -> Column_4(1B)/1
  Byte_06/1 -> Column_7(1B)/1
  Byte_1/1 -> Column_1(1B)/1
  Byte_02/1 -> Column_3(1B)/1

== system Pokus07_Display/Character_Table/Characters(0..F)/Char_5 ==
  Byte_01 : Constant  Value=char(:, 2, 5)  OutDataTypeStr=uint8
  Byte_02 : Constant  Value=char(:, 3, 5)  OutDataTypeStr=uint8
  Byte_03 : Constant  Value=char(:, 4, 5)  OutDataTypeStr=uint8
  Byte_04 : Constant  Value=char(:, 5, 5)  OutDataTypeStr=uint8
  Byte_05 : Constant  Value=char(:, 6, 5)  OutDataTypeStr=uint8
  Byte_06 : Constant  Value=char(:, 7, 5)  OutDataTypeStr=uint8
  Byte_07 : Constant  Value=char(:, 8, 5)  OutDataTypeStr=uint8
  Byte_1 : Constant  Value=char(:, 1, 5)  OutDataTypeStr=uint8
  Column_1(1B) : Outport
  Column_2(1B) : Outport  Port=2
  Column_3(1B) : Outport  Port=3
  Column_4(1B) : Outport  Port=4
  Column_5(1B) : Outport  Port=5
  Column_6(1B) : Outport  Port=6
  Column_7(1B) : Outport  Port=7
  Column_8(1B) : Outport  Port=8
  wires:
  Byte_05/1 -> Column_6(1B)/1
  Byte_04/1 -> Column_5(1B)/1
  Byte_01/1 -> Column_2(1B)/1
  Byte_07/1 -> Column_8(1B)/1
  Byte_03/1 -> Column_4(1B)/1
  Byte_06/1 -> Column_7(1B)/1
  Byte_1/1 -> Column_1(1B)/1
  Byte_02/1 -> Column_3(1B)/1

== system Pokus07_Display/Character_Table/Characters(0..F)/Char_6 ==
  Byte_01 : Constant  Value=char(:, 2, 6)  OutDataTypeStr=uint8
  Byte_02 : Constant  Value=char(:, 3, 6)  OutDataTypeStr=uint8
  Byte_03 : Constant  Value=char(:, 4, 6)  OutDataTypeStr=uint8
  Byte_04 : Constant  Value=char(:, 5, 6)  OutDataTypeStr=uint8
  Byte_05 : Constant  Value=char(:, 6, 6)  OutDataTypeStr=uint8
  Byte_06 : Constant  Value=char(:, 7, 6)  OutDataTypeStr=uint8
  Byte_07 : Constant  Value=char(:, 8, 6)  OutDataTypeStr=uint8
  Byte_1 : Constant  Value=char(:, 1, 6)  OutDataTypeStr=uint8
  Column_1(1B) : Outport
  Column_2(1B) : Outport  Port=2
  Column_3(1B) : Outport  Port=3
  Column_4(1B) : Outport  Port=4
  Column_5(1B) : Outport  Port=5
  Column_6(1B) : Outport  Port=6
  Column_7(1B) : Outport  Port=7
  Column_8(1B) : Outport  Port=8
  wires:
  Byte_05/1 -> Column_6(1B)/1
  Byte_04/1 -> Column_5(1B)/1
  Byte_01/1 -> Column_2(1B)/1
  Byte_07/1 -> Column_8(1B)/1
  Byte_03/1 -> Column_4(1B)/1
  Byte_06/1 -> Column_7(1B)/1
  Byte_1/1 -> Column_1(1B)/1
  Byte_02/1 -> Column_3(1B)/1

== system Pokus07_Display/Character_Table/Characters(0..F)/Char_7 ==
  Byte_01 : Constant  Value=char(:, 2, 7)  OutDataTypeStr=uint8
  Byte_02 : Constant  Value=char(:, 3, 7)  OutDataTypeStr=uint8
  Byte_03 : Constant  Value=char(:, 4, 7)  OutDataTypeStr=uint8
  Byte_04 : Constant  Value=char(:, 5, 7)  OutDataTypeStr=uint8
  Byte_05 : Constant  Value=char(:, 6, 7)  OutDataTypeStr=uint8
  Byte_06 : Constant  Value=char(:, 7, 7)  OutDataTypeStr=uint8
  Byte_07 : Constant  Value=char(:, 8, 7)  OutDataTypeStr=uint8
  Byte_1 : Constant  Value=char(:, 1, 7)  OutDataTypeStr=uint8
  Column_1(1B) : Outport
  Column_2(1B) : Outport  Port=2
  Column_3(1B) : Outport  Port=3
  Column_4(1B) : Outport  Port=4
  Column_5(1B) : Outport  Port=5
  Column_6(1B) : Outport  Port=6
  Column_7(1B) : Outport  Port=7
  Column_8(1B) : Outport  Port=8
  wires:
  Byte_05/1 -> Column_6(1B)/1
  Byte_04/1 -> Column_5(1B)/1
  Byte_01/1 -> Column_2(1B)/1
  Byte_07/1 -> Column_8(1B)/1
  Byte_03/1 -> Column_4(1B)/1
  Byte_06/1 -> Column_7(1B)/1
  Byte_1/1 -> Column_1(1B)/1
  Byte_02/1 -> Column_3(1B)/1

== system Pokus07_Display/Character_Table/Characters(0..F)/Char_8 ==
  Byte_01 : Constant  Value=char(:, 2, 8)  OutDataTypeStr=uint8
  Byte_02 : Constant  Value=char(:, 3, 8)  OutDataTypeStr=uint8
  Byte_03 : Constant  Value=char(:, 4, 8)  OutDataTypeStr=uint8
  Byte_04 : Constant  Value=char(:, 5, 8)  OutDataTypeStr=uint8
  Byte_05 : Constant  Value=char(:, 6, 8)  OutDataTypeStr=uint8
  Byte_06 : Constant  Value=char(:, 7, 8)  OutDataTypeStr=uint8
  Byte_07 : Constant  Value=char(:, 8, 8)  OutDataTypeStr=uint8
  Byte_1 : Constant  Value=char(:, 1, 8)  OutDataTypeStr=uint8
  Column_1(1B) : Outport
  Column_2(1B) : Outport  Port=2
  Column_3(1B) : Outport  Port=3
  Column_4(1B) : Outport  Port=4
  Column_5(1B) : Outport  Port=5
  Column_6(1B) : Outport  Port=6
  Column_7(1B) : Outport  Port=7
  Column_8(1B) : Outport  Port=8
  wires:
  Byte_05/1 -> Column_6(1B)/1
  Byte_04/1 -> Column_5(1B)/1
  Byte_01/1 -> Column_2(1B)/1
  Byte_07/1 -> Column_8(1B)/1
  Byte_03/1 -> Column_4(1B)/1
  Byte_06/1 -> Column_7(1B)/1
  Byte_1/1 -> Column_1(1B)/1
  Byte_02/1 -> Column_3(1B)/1

== system Pokus07_Display/Character_Table/Characters(0..F)/Char_9 ==
  Byte_01 : Constant  Value=char(:, 2, 9)  OutDataTypeStr=uint8
  Byte_02 : Constant  Value=char(:, 3, 9)  OutDataTypeStr=uint8
  Byte_03 : Constant  Value=char(:, 4, 9)  OutDataTypeStr=uint8
  Byte_04 : Constant  Value=char(:, 5, 9)  OutDataTypeStr=uint8
  Byte_05 : Constant  Value=char(:, 6, 9)  OutDataTypeStr=uint8
  Byte_06 : Constant  Value=char(:, 7, 9)  OutDataTypeStr=uint8
  Byte_07 : Constant  Value=char(:, 8, 9)  OutDataTypeStr=uint8
  Byte_1 : Constant  Value=char(:, 1, 9)  OutDataTypeStr=uint8
  Column_1(1B) : Outport
  Column_2(1B) : Outport  Port=2
  Column_3(1B) : Outport  Port=3
  Column_4(1B) : Outport  Port=4
  Column_5(1B) : Outport  Port=5
  Column_6(1B) : Outport  Port=6
  Column_7(1B) : Outport  Port=7
  Column_8(1B) : Outport  Port=8
  wires:
  Byte_05/1 -> Column_6(1B)/1
  Byte_04/1 -> Column_5(1B)/1
  Byte_01/1 -> Column_2(1B)/1
  Byte_07/1 -> Column_8(1B)/1
  Byte_03/1 -> Column_4(1B)/1
  Byte_06/1 -> Column_7(1B)/1
  Byte_1/1 -> Column_1(1B)/1
  Byte_02/1 -> Column_3(1B)/1

== system Pokus07_Display/Character_Table/Characters(0..F)/Char_A ==
  Byte_01 : Constant  Value=char(:, 2, A)  OutDataTypeStr=uint8
  Byte_02 : Constant  Value=char(:, 3, A)  OutDataTypeStr=uint8
  Byte_03 : Constant  Value=char(:, 4, A)  OutDataTypeStr=uint8
  Byte_04 : Constant  Value=char(:, 5, A)  OutDataTypeStr=uint8
  Byte_05 : Constant  Value=char(:, 6, A)  OutDataTypeStr=uint8
  Byte_06 : Constant  Value=char(:, 7, A)  OutDataTypeStr=uint8
  Byte_07 : Constant  Value=char(:, 8, A)  OutDataTypeStr=uint8
  Byte_1 : Constant  Value=char(:, 1, A)  OutDataTypeStr=uint8
  Column_1(1B) : Outport
  Column_2(1B) : Outport  Port=2
  Column_3(1B) : Outport  Port=3
  Column_4(1B) : Outport  Port=4
  Column_5(1B) : Outport  Port=5
  Column_6(1B) : Outport  Port=6
  Column_7(1B) : Outport  Port=7
  Column_8(1B) : Outport  Port=8
  wires:
  Byte_05/1 -> Column_6(1B)/1
  Byte_04/1 -> Column_5(1B)/1
  Byte_01/1 -> Column_2(1B)/1
  Byte_07/1 -> Column_8(1B)/1
  Byte_03/1 -> Column_4(1B)/1
  Byte_06/1 -> Column_7(1B)/1
  Byte_1/1 -> Column_1(1B)/1
  Byte_02/1 -> Column_3(1B)/1

== system Pokus07_Display/Character_Table/Characters(0..F)/Char_B ==
  Byte_01 : Constant  Value=char(:, 2, B)  OutDataTypeStr=uint8
  Byte_02 : Constant  Value=char(:, 3, B)  OutDataTypeStr=uint8
  Byte_03 : Constant  Value=char(:, 4, B)  OutDataTypeStr=uint8
  Byte_04 : Constant  Value=char(:, 5, B)  OutDataTypeStr=uint8
  Byte_05 : Constant  Value=char(:, 6, B)  OutDataTypeStr=uint8
  Byte_06 : Constant  Value=char(:, 7, B)  OutDataTypeStr=uint8
  Byte_07 : Constant  Value=char(:, 8, B)  OutDataTypeStr=uint8
  Byte_1 : Constant  Value=char(:, 1, B)  OutDataTypeStr=uint8
  Column_1(1B) : Outport
  Column_2(1B) : Outport  Port=2
  Column_3(1B) : Outport  Port=3
  Column_4(1B) : Outport  Port=4
  Column_5(1B) : Outport  Port=5
  Column_6(1B) : Outport  Port=6
  Column_7(1B) : Outport  Port=7
  Column_8(1B) : Outport  Port=8
  wires:
  Byte_05/1 -> Column_6(1B)/1
  Byte_04/1 -> Column_5(1B)/1
  Byte_01/1 -> Column_2(1B)/1
  Byte_07/1 -> Column_8(1B)/1
  Byte_03/1 -> Column_4(1B)/1
  Byte_06/1 -> Column_7(1B)/1
  Byte_1/1 -> Column_1(1B)/1
  Byte_02/1 -> Column_3(1B)/1

== system Pokus07_Display/Character_Table/Characters(0..F)/Char_C ==
  Byte_01 : Constant  Value=char(:, 2, C)  OutDataTypeStr=uint8
  Byte_02 : Constant  Value=char(:, 3, C)  OutDataTypeStr=uint8
  Byte_03 : Constant  Value=char(:, 4, C)  OutDataTypeStr=uint8
  Byte_04 : Constant  Value=char(:, 5, C)  OutDataTypeStr=uint8
  Byte_05 : Constant  Value=char(:, 6, C)  OutDataTypeStr=uint8
  Byte_06 : Constant  Value=char(:, 7, C)  OutDataTypeStr=uint8
  Byte_07 : Constant  Value=char(:, 8, C)  OutDataTypeStr=uint8
  Byte_1 : Constant  Value=char(:, 1, C)  OutDataTypeStr=uint8
  Column_1(1B) : Outport
  Column_2(1B) : Outport  Port=2
  Column_3(1B) : Outport  Port=3
  Column_4(1B) : Outport  Port=4
  Column_5(1B) : Outport  Port=5
  Column_6(1B) : Outport  Port=6
  Column_7(1B) : Outport  Port=7
  Column_8(1B) : Outport  Port=8
  wires:
  Byte_05/1 -> Column_6(1B)/1
  Byte_04/1 -> Column_5(1B)/1
  Byte_01/1 -> Column_2(1B)/1
  Byte_07/1 -> Column_8(1B)/1
  Byte_03/1 -> Column_4(1B)/1
  Byte_06/1 -> Column_7(1B)/1
  Byte_1/1 -> Column_1(1B)/1
  Byte_02/1 -> Column_3(1B)/1

== system Pokus07_Display/Character_Table/Characters(0..F)/Char_D ==
  Byte_01 : Constant  Value=char(:, 2, D)  OutDataTypeStr=uint8
  Byte_02 : Constant  Value=char(:, 3, D)  OutDataTypeStr=uint8
  Byte_03 : Constant  Value=char(:, 4, D)  OutDataTypeStr=uint8
  Byte_04 : Constant  Value=char(:, 5, D)  OutDataTypeStr=uint8
  Byte_05 : Constant  Value=char(:, 6, D)  OutDataTypeStr=uint8
  Byte_06 : Constant  Value=char(:, 7, D)  OutDataTypeStr=uint8
  Byte_07 : Constant  Value=char(:, 8, D)  OutDataTypeStr=uint8
  Byte_1 : Constant  Value=char(:, 1, D)  OutDataTypeStr=uint8
  Column_1(1B) : Outport
  Column_2(1B) : Outport  Port=2
  Column_3(1B) : Outport  Port=3
  Column_4(1B) : Outport  Port=4
  Column_5(1B) : Outport  Port=5
  Column_6(1B) : Outport  Port=6
  Column_7(1B) : Outport  Port=7
  Column_8(1B) : Outport  Port=8
  wires:
  Byte_05/1 -> Column_6(1B)/1
  Byte_04/1 -> Column_5(1B)/1
  Byte_01/1 -> Column_2(1B)/1
  Byte_07/1 -> Column_8(1B)/1
  Byte_03/1 -> Column_4(1B)/1
  Byte_06/1 -> Column_7(1B)/1
  Byte_1/1 -> Column_1(1B)/1
  Byte_02/1 -> Column_3(1B)/1

== system Pokus07_Display/Character_Table/Characters(0..F)/Char_E ==
  Byte_01 : Constant  Value=char(:, 2, E)  OutDataTypeStr=uint8
  Byte_02 : Constant  Value=char(:, 3, E)  OutDataTypeStr=uint8
  Byte_03 : Constant  Value=char(:, 4, E)  OutDataTypeStr=uint8
  Byte_04 : Constant  Value=char(:, 5, E)  OutDataTypeStr=uint8
  Byte_05 : Constant  Value=char(:, 6, E)  OutDataTypeStr=uint8
  Byte_06 : Constant  Value=char(:, 7, E)  OutDataTypeStr=uint8
  Byte_07 : Constant  Value=char(:, 8, E)  OutDataTypeStr=uint8
  Byte_1 : Constant  Value=char(:, 1, E)  OutDataTypeStr=uint8
  Column_1(1B) : Outport
  Column_2(1B) : Outport  Port=2
  Column_3(1B) : Outport  Port=3
  Column_4(1B) : Outport  Port=4
  Column_5(1B) : Outport  Port=5
  Column_6(1B) : Outport  Port=6
  Column_7(1B) : Outport  Port=7
  Column_8(1B) : Outport  Port=8
  wires:
  Byte_05/1 -> Column_6(1B)/1
  Byte_04/1 -> Column_5(1B)/1
  Byte_01/1 -> Column_2(1B)/1
  Byte_07/1 -> Column_8(1B)/1
  Byte_03/1 -> Column_4(1B)/1
  Byte_06/1 -> Column_7(1B)/1
  Byte_1/1 -> Column_1(1B)/1
  Byte_02/1 -> Column_3(1B)/1

== system Pokus07_Display/Character_Table/Characters(0..F)/Char_F ==
  Byte_01 : Constant  Value=char(:, 2, F)  OutDataTypeStr=uint8
  Byte_02 : Constant  Value=char(:, 3, F)  OutDataTypeStr=uint8
  Byte_03 : Constant  Value=char(:, 4, F)  OutDataTypeStr=uint8
  Byte_04 : Constant  Value=char(:, 5, F)  OutDataTypeStr=uint8
  Byte_05 : Constant  Value=char(:, 6, F)  OutDataTypeStr=uint8
  Byte_06 : Constant  Value=char(:, 7, F)  OutDataTypeStr=uint8
  Byte_07 : Constant  Value=char(:, 8, F)  OutDataTypeStr=uint8
  Byte_1 : Constant  Value=char(:, 1, F)  OutDataTypeStr=uint8
  Column_1(1B) : Outport
  Column_2(1B) : Outport  Port=2
  Column_3(1B) : Outport  Port=3
  Column_4(1B) : Outport  Port=4
  Column_5(1B) : Outport  Port=5
  Column_6(1B) : Outport  Port=6
  Column_7(1B) : Outport  Port=7
  Column_8(1B) : Outport  Port=8
  wires:
  Byte_05/1 -> Column_6(1B)/1
  Byte_04/1 -> Column_5(1B)/1
  Byte_01/1 -> Column_2(1B)/1
  Byte_07/1 -> Column_8(1B)/1
  Byte_03/1 -> Column_4(1B)/1
  Byte_06/1 -> Column_7(1B)/1
  Byte_1/1 -> Column_1(1B)/1
  Byte_02/1 -> Column_3(1B)/1

== system Pokus07_Display/Character_Table/Characters(ARROW_DOWN..RECTANGLE)/Char_ARROW_DOWN ==
  Byte_01 : Constant  Value=char(2, ARROW_DOWN)  OutDataTypeStr=uint8
  Byte_02 : Constant  Value=char(3, ARROW_DOWN)  OutDataTypeStr=uint8
  Byte_03 : Constant  Value=char(4, ARROW_DOWN)  OutDataTypeStr=uint8
  Byte_04 : Constant  Value=char(5, ARROW_DOWN)  OutDataTypeStr=uint8
  Byte_05 : Constant  Value=char(6, ARROW_DOWN)  OutDataTypeStr=uint8
  Byte_06 : Constant  Value=char(7, ARROW_DOWN)  OutDataTypeStr=uint8
  Byte_07 : Constant  Value=char(8, ARROW_DOWN)  OutDataTypeStr=uint8
  Byte_1 : Constant  Value=char(1, ARROW_DOWN)  OutDataTypeStr=uint8
  Column_1(1B) : Outport
  Column_2(1B) : Outport  Port=2
  Column_3(1B) : Outport  Port=3
  Column_4(1B) : Outport  Port=4
  Column_5(1B) : Outport  Port=5
  Column_6(1B) : Outport  Port=6
  Column_7(1B) : Outport  Port=7
  Column_8(1B) : Outport  Port=8
  wires:
  Byte_05/1 -> Column_6(1B)/1
  Byte_04/1 -> Column_5(1B)/1
  Byte_01/1 -> Column_2(1B)/1
  Byte_07/1 -> Column_8(1B)/1
  Byte_03/1 -> Column_4(1B)/1
  Byte_06/1 -> Column_7(1B)/1
  Byte_1/1 -> Column_1(1B)/1
  Byte_02/1 -> Column_3(1B)/1
